simulink model "modelo2a"  (R2024b)
settings: Solver=ode4  StartTime=0.0  StopTime=t_final  FixedStep=t_step  RelTol=1e-3  EnableMultiTasking=on
InitFcn:
  | modelo2Initialization
undefined symbols (not defined in the file): Earth, IC, Quadrotor, sigbuilder_block, t_step, WGS84
libraries: simulink_extras x2, aerolibfltsims x2, aerolibobsolete x1, aerolibtransform2 x1, aerolibanimutils x1
settings Model: Creator=claus  LastModifiedBy=krish
settings SolverCC: ShapePreserveControl=EnableAll  AlgebraicLoopSolver=TrustRegion
settings DataIOCC: LimitDataPoints=on  SaveFormat=Array  ReturnWorkspaceOutputs=off
settings OptimizationCC: ExpressionDepthLimit=2147483647  EfficientMapNaN2IntZero=off  LifeSpan=inf  SimCompilerOptimization=on  AccelVerboseBuild=on
settings DebuggingCC: UnderspecifiedInitializationDetection=Classic  MergeDetectMultiDrivingBlocksExec=none  SolverPrmCheckMsg=warning  UnconnectedInputMsg=warning  UnconnectedOutputMsg=warning  UnconnectedLineMsg=warning  StateNameClashWarn=warning  SFUnexpectedBacktrackingDiag=warning  SFNoUnconditionalDefaultTransitionDiag=warning  SFExecutionAtInitializationDiag=none  ArithmeticOperatorsInVariantConditions=warning
settings HardwareCC: ProdBitPerPointer=32  ProdBitPerSizeT=32  ProdBitPerPtrDiffT=32  ProdLargestAtomicFloat=None  ProdIntDivRoundTo=Undefined  ProdEndianess=Unspecified  ProdWordSize=32  ProdHWDeviceType=32-bit Generic  TargetBitPerPointer=64  TargetBitPerSizeT=64  TargetBitPerPtrDiffT=64  TargetLongLongMode=on  TargetIntDivRoundTo=Zero  TargetEndianess=LittleEndian  TargetWordSize=64  TargetHWDeviceType=MATLAB Host  ProdEqTarget=off
settings ModelReferenceCC: EnableParallelModelReferenceBuilds=on  PropagateSignalLabelsOutOfModel=off
settings SFSimCC: SimUseLocalCustomCode=off  CustomCodeUndefinedFunction=UseInterfaceOnly
settings RTWCC: RTWUseLocalCustomCode=off  GPUComputeCapability=3.5
settings CodeAppCC: MaxIdLength=128  StateflowObjectComments=on
settings GRTTargetCC: TargetLangStandard=C89/C90 (ANSI)  CombineOutputUpdateFcns=off  GRTInterface=on
settings ConfigComp: CovMetricSettings=dw  CovSaveCumulativeToWorkspaceVar=on  CovSaveSingleToWorkspaceVar=on  CovExternalEMLEnable=off

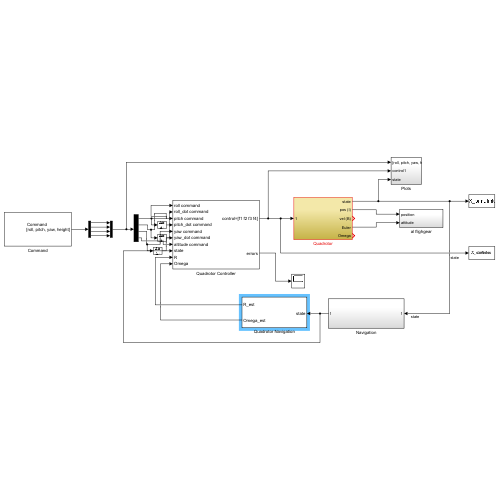
[thumbnail: Simulink's stored preview of the top-level diagram]
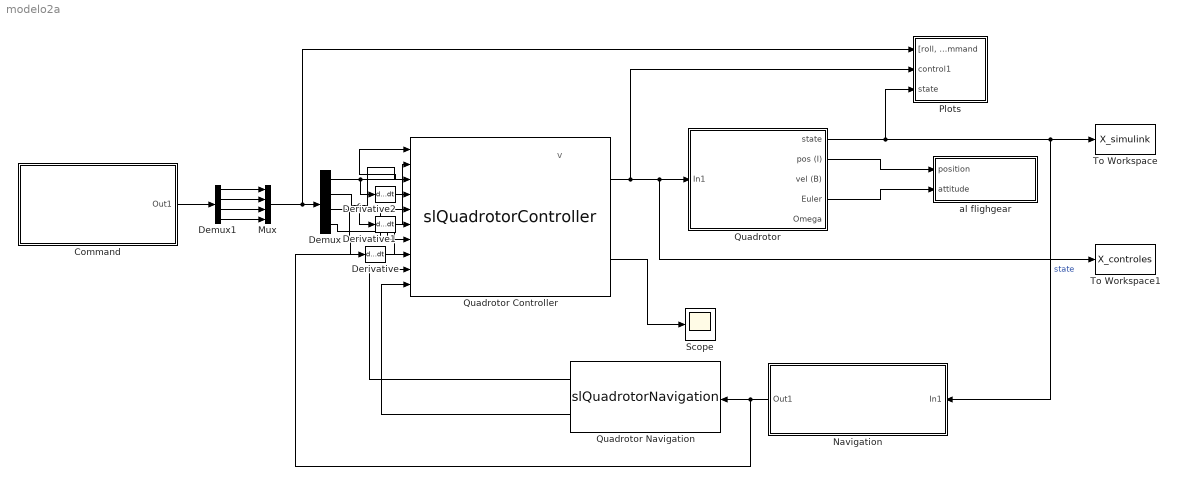
== system modelo2a ==
  note: v
  Command : Subsystem
      mask Display:
      | fprintf('Command \n \n')
      | port_label('output', 1, '[roll, pitch, yaw, height]')
  Demux : Demux
  Demux1 : Demux
  Derivative : Derivative
  Derivative1 : Derivative
  Derivative2 : Derivative
  Mux : Mux
  Navigation : Subsystem
  Plots : Subsystem
  Quadrotor : Subsystem
  Quadrotor Controller : M-S-Function  FunctionName=slQuadrotorController
      mask Display:
      | port_label('output', 1, 'control=[f1 f2 f3 f4]')
      | port_label('output', 2, 'errors')
      | port_label('input', 1, 'roll command')
      | port_label('input', 3, 'pitch command')
      | port_label('input', 5, 'yaw command')
      | port_label('input', 2, 'roll_dot command')
      | port_label('input', 4, 'pitch_dot command')
      | port_label('input', 6, 'yaw_dot command')
      | port_label('input', 7, 'altitude command')
      | port_label('input', 8, 'state')
      | port_label('input', 9, 'R')
      | port_label('input', 10, 'Omega')
  "Quadrotor Navigation " : M-S-Function  FunctionName=slQuadrotorNavigation
      mask Display:
      | port_label('output', 1, 'R_est')
      | port_label('output', 2, 'Omega_est')
      | port_label('input', 1, 'state')
  Scope : Scope
  To Workspace : ToWorkspace  VariableName=X_simulink  SaveFormat=Timeseries  SampleTime=-1
  To Workspace1 : ToWorkspace  VariableName=X_controles  SaveFormat=Timeseries  SampleTime=-1
  al flighgear : Subsystem
  wires:
  Quadrotor Controller/1 -> To Workspace1/1, Quadrotor/1(In1), Plots/2(control1)
  Quadrotor/1(state) -> Navigation/1(In1), To Workspace/1, Plots/3(state)  "state"
  Quadrotor/2(pos (I)) -> al flighgear/1(position)
  Quadrotor/4(Euler) -> al flighgear/2(attitude)
  Mux/1 -> Demux/1, Plots/1("[roll, pitch, yaw, height] command")
  Demux/1 -> Derivative2/1, Quadrotor Controller/1
  Demux/2 -> Derivative1/1, Quadrotor Controller/3
  Demux/3 -> Derivative/1, Quadrotor Controller/5
  Demux/4 -> Quadrotor Controller/7
  Derivative/1 -> Quadrotor Controller/6
  Derivative1/1 -> Quadrotor Controller/4
  Derivative2/1 -> Quadrotor Controller/2
  Command/1(Out1) -> Demux1/1
  Demux1/2 -> Mux/2
  "Quadrotor Navigation "/1 -> Quadrotor Controller/9
  "Quadrotor Navigation "/2 -> Quadrotor Controller/10
  Navigation/1(Out1) -> Quadrotor Controller/8, "Quadrotor Navigation "/1
  Quadrotor Controller/2 -> Scope/1
  Demux1/1 -> Mux/1
  Demux1/4 -> Mux/4
  Demux1/3 -> Mux/3

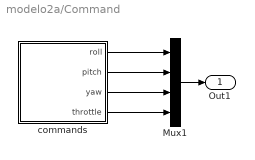
== system modelo2a/Command ==
  Mux1 : Mux
  commands : Subsystem  Tag=STV Subsys  LoadFcn=sigbuilder_block('load',[0 36 960 449.5 ]);  StartFcn=sigbuilder_block('start');  StopFcn=sigbuilder_block('stop');  ClipboardFcn=sigbuilder_block('clipboard');  mask(Sigbuilder block){tuvar=[0:10]}
      mask help: Simulink:masks:SigbuilderBlock_MD
      mask init:
      | if ~strcmp(get_param(bdroot(gcbh),'SimulationStatus'),'stopped') tuvar = sigbuilder_block('maskInit'); end
      settings: CopyFcn=sigbuilder_block('copy');  DeleteFcn=sigbuilder_block('delete');  ModelCloseFcn=sigbuilder_block('modelClose');  PreSaveFcn=sigbuilder_block('preSave');  PauseFcn=sigbuilder_block('pause');  ContinueFcn=sigbuilder_block('continue');  NameChangeFcn=sigbuilder_block('namechange');  OpenFcn=sigbuilder_block('open',[110.618 111.614 951.71 513.226 ]);  CloseFcn=sigbuilder_block('close');
      mask Display: plot(0, 0, 100, 100,[2, 2, 32, 32, 2], [68, 8, 8, 68, 68],[32, 2], [38, 38], [32, 19, 2],[53, 60, 44], [32, 17, 17, 2],[16, 16, 31, 31]);txt = getActiveGroup(gcbh);text(2, 100, txt,'verticalAlignment', 'top');
  Out1 : Outport
  wires:
  commands/1(roll) -> Mux1/1
  commands/2(pitch) -> Mux1/2
  commands/3(yaw) -> Mux1/3
  commands/4(throttle) -> Mux1/4
  Mux1/1 -> Out1/1

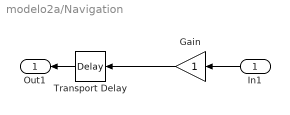
== system modelo2a/Navigation ==
  In1 : Inport
  Gain : Gain
  Transport Delay : TransportDelay  DelayTime=t_step*1
  Out1 : Outport
  wires:
  Gain/1 -> Transport Delay/1
  In1/1 -> Gain/1
  Transport Delay/1 -> Out1/1

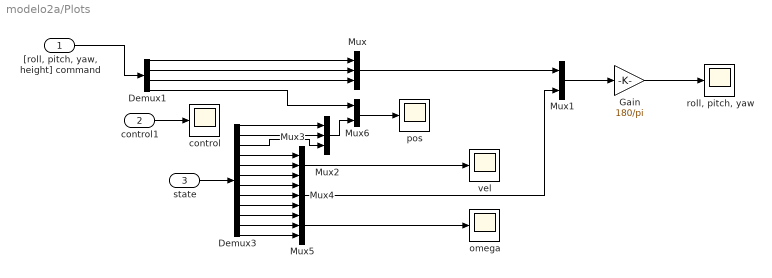
== system modelo2a/Plots ==
  "[roll, pitch, yaw, height] command" : Inport
  control1 : Inport  Port=2
  state : Inport  Port=3
  Demux1 : Demux
  Demux3 : Demux  Outputs=12
  Gain : Gain  Gain=180/pi
  Mux{,2..5} (5 alike) : Mux  Inputs=3
  Mux1 : Mux  Inputs=2
  Mux6 : Mux  Inputs=2
  control : Scope
  omega : Scope
  pos : Scope
  "roll, pitch, yaw" : Scope
  vel : Scope
  wires:
  Mux/1 -> Mux1/1
  Mux1/1 -> Gain/1
  Demux3/1 -> Mux2/1
  Demux3/2 -> Mux2/2
  Demux3/3 -> Mux2/3
  Demux3/4 -> Mux3/1
  Demux3/5 -> Mux3/2
  Demux3/6 -> Mux3/3
  Demux3/7 -> Mux4/1
  Demux3/8 -> Mux4/2
  Demux3/9 -> Mux4/3
  Demux3/10 -> Mux5/1
  Demux3/11 -> Mux5/2
  Demux3/12 -> Mux5/3
  Mux4/1 -> Mux1/2
  Mux6/1 -> pos/1
  Mux2/1 -> Mux6/2
  Mux5/1 -> omega/1
  Mux3/1 -> vel/1
  "[roll, pitch, yaw, height] command"/1 -> Demux1/1
  control1/1 -> control/1
  state/1 -> Demux3/1
  Demux1/4 -> Mux6/1
  Demux1/1 -> Mux/1
  Demux1/3 -> Mux/3
  Demux1/2 -> Mux/2
  Gain/1 -> "roll, pitch, yaw"/1

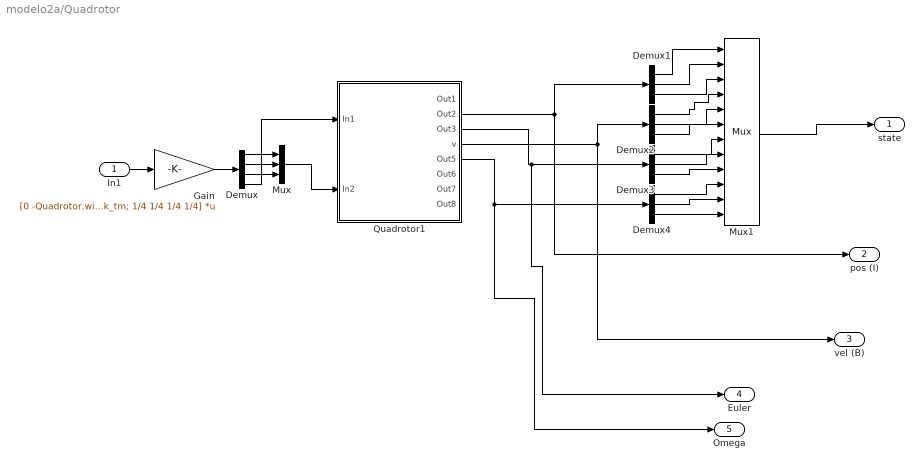
== system modelo2a/Quadrotor ==
  In1 : Inport
  Demux : Demux
  Demux{1..4} (4 alike) : Demux  Outputs=3
  Gain : Gain  Gain=[0 -Quadrotor.width/2 0 Quadrotor.width/2; -Quadrotor.width/2 0 Quadrotor.width/2 0; Quadrotor.k_tm -Quadrotor.k_tm Quadrotor.k_tm -Quadrotor.k_tm; 1/4 1/4 1/4 1/4]  Multiplication=Matrix(K*u)
  Mux : Mux  Inputs=3
  Mux1 : Mux  Inputs=12
  Quadrotor1 : Subsystem
      mask Display:
      | port_label('input', 1, 'Fz')
      | port_label('input', 2, 'Mxyz')
      | port_label('output', 2, 'r')
      | port_label('output', 3, 'Euler')
      | port_label('output', 4, 'v')
      | port_label('output', 5, 'Omega')
      | port_label('output', 8, 'R')
  state : Outport
  pos (I) : Outport  Port=2
  vel (B) : Outport  Port=3
  Euler : Outport  Port=4
  Omega : Outport  Port=5
  wires:
  Gain/1 -> Demux/1
  Mux/1 -> Quadrotor1/2(In2)
  Quadrotor1/4(v) -> vel (B)/1, Demux2/1
  Quadrotor1/3(Out3) -> Euler/1, Demux3/1
  Quadrotor1/5(Out5) -> Omega/1, Demux4/1
  Demux1/3 -> Mux1/3
  Demux1/2 -> Mux1/2
  Demux1/1 -> Mux1/1
  Demux2/1 -> Mux1/4
  Demux2/2 -> Mux1/5
  Demux2/3 -> Mux1/6
  Demux3/1 -> Mux1/7
  Demux3/2 -> Mux1/8
  Demux3/3 -> Mux1/9
  Demux4/1 -> Mux1/10
  Demux4/2 -> Mux1/11
  Demux4/3 -> Mux1/12
  Mux1/1 -> state/1
  Quadrotor1/2(Out2) -> pos (I)/1, Demux1/1
  In1/1 -> Gain/1
  Demux/2 -> Mux/2
  Demux/3 -> Mux/3
  Demux/1 -> Mux/1
  Demux/4 -> Quadrotor1/1(In1)

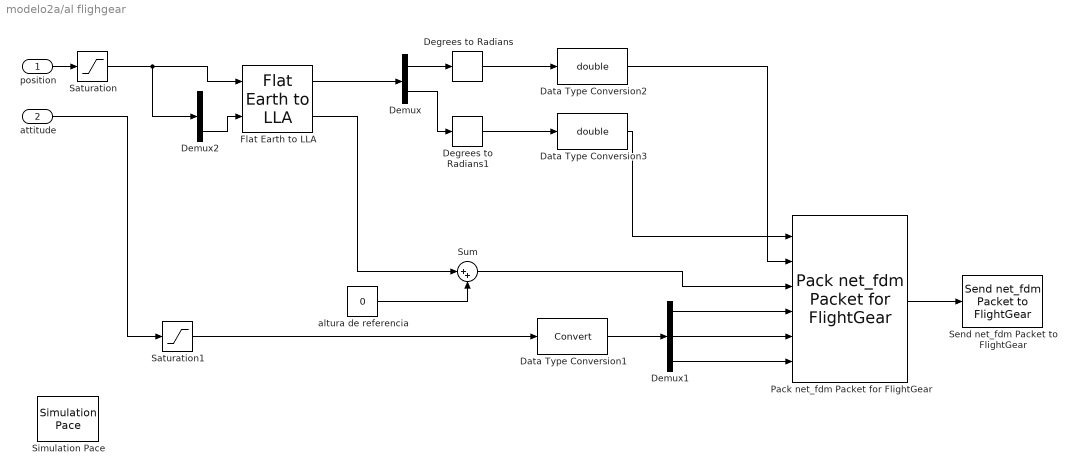
== system modelo2a/al flighgear ==
  position : Inport
  attitude : Inport  Port=2
  Data Type Conversion1 : DataTypeConversion  SaturateOnIntegerOverflow=off  RndMeth=Floor
  Data Type Conversion2 : DataTypeConversion  OutDataTypeStr=double  SaturateOnIntegerOverflow=off  RndMeth=Floor
  Data Type Conversion3 : DataTypeConversion  OutDataTypeStr=double  SaturateOnIntegerOverflow=off  RndMeth=Floor
  Degrees to Radians : simulink_extras/Transformations/Degrees to Radians
  Degrees to Radians1 : simulink_extras/Transformations/Degrees to Radians
  Demux : Demux  Outputs=2
  Demux1 : Demux  Outputs=3
  Demux2 : Demux  Outputs=3
  Flat Earth to LLA : aerolibtransform2/Flat Earth to LLA  units=Metric (MKS)  ptype=Earth (WGS84)  F=1/298.257223563  R=6378137  refPosPort=off  LL0=IC.LatLonAltOnEarth(1:2)  psi=0
  Pack net_fdm Packet for FlightGear : aerolibfltsims/Pack net_fdm Packet for FlightGear  FlightGearVersion=v2.8  ShowPositionAttitudeInputs=on  ShowVelocityAccelerationInputs=off  ShowControlSurfacePositionInputs=off  ShowEngineFuelInputs=off  ShowLandingGearInputs=off  ShowEnvironmentInputs=off  SampleTime=-1  packetVersion=24
  Saturation : Saturate  UpperLimit=100  LowerLimit=-100
  Saturation1 : Saturate  UpperLimit=100  LowerLimit=-100
  Send net_fdm Packet to FlightGear : aerolibfltsims/Send net_fdm Packet to FlightGear  DestinationIpAddress=127.0.0.1  DestinationPort=5502  LocalIpPort=-1  varLen=off  SampleTime=-1
  Simulation Pace : aerolibanimutils/Simulation Pace  SimulationPace=1  SleepMode=MATLAB Thread  OutputPaceError=off  SampleTime=-1
      settings: AttributesFormatString=%<SimulationPace> sec/sec
  Sum : Sum  Inputs=|++
  altura de referencia : Constant  Value=0
  wires:
  position/1 -> Saturation/1
  attitude/1 -> Saturation1/1
  Pack net_fdm Packet for FlightGear/1 -> Send net_fdm Packet to FlightGear/1
  Demux1/1 -> Pack net_fdm Packet for FlightGear/4
  Demux1/2 -> Pack net_fdm Packet for FlightGear/5
  Demux1/3 -> Pack net_fdm Packet for FlightGear/6
  Data Type Conversion1/1 -> Demux1/1
  Flat Earth to LLA/1 -> Demux/1
  Demux2/3 -> Flat Earth to LLA/2
  Degrees to Radians/1 -> Data Type Conversion2/1
  Degrees to Radians1/1 -> Data Type Conversion3/1
  Demux/1 -> Degrees to Radians/1
  Demux/2 -> Degrees to Radians1/1
  Data Type Conversion3/1 -> Pack net_fdm Packet for FlightGear/1
  Data Type Conversion2/1 -> Pack net_fdm Packet for FlightGear/2
  Flat Earth to LLA/2 -> Sum/1
  altura de referencia/1 -> Sum/2
  Sum/1 -> Pack net_fdm Packet for FlightGear/3
  Saturation/1 -> Demux2/1, Flat Earth to LLA/1
  Saturation1/1 -> Data Type Conversion1/1

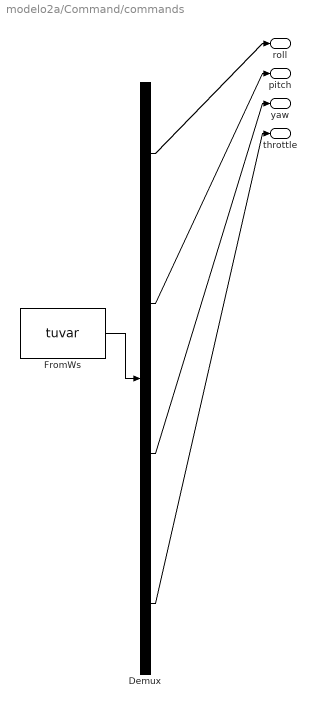
== system modelo2a/Command/commands ==
  Demux : Demux  Tag=STV Demux
      settings: DisplayOption=none
  FromWs : FromWorkspace  Tag=STV FromWs  VariableName=tuvar
      SigBuilderData=|
      | common.afterFinalStr = 'Extrapolate'
      | common.sampleTime = 0
      | dataSet.timeRange = [0 15]
      | dataSet.name = 'Group 1'
      | sbobj.Groups.Name = 'Group 1'
      | sbobj.Groups.Signals(1).Name = 'roll'
      | sbobj.Groups.Signals(1).XData = [0 1 2 2 6 6 7 11 12 15]
      | sbobj.Groups.Signals(1).YData = [0 0 6.28 6.3 6.3 6.28 -0.3 -0.3 0 0]
      | sbobj.Groups.Signals(2).Name = 'pitch'
      | sbobj.Groups.Signals(2).XData = [0 1 5 11.4 15]
      | sbobj.Groups.Signals(2).YData = [0 0 0 0 0]
      | sbobj.Groups.Signals(3).Name = 'yaw'
      | sbobj.Groups.Signals(3).XData = [0 0.6 3.45 5 6.5 8.5 15]
      | sbobj.Groups.Signals(3).YData = [0 0 0 0 0 0 0]
      | sbobj.Groups.Signals(4).Name = 'throttle'
      | sbobj.Groups.Signals(4).XData = [0 0.94 1 2.94 2.94 5.8 5.8 11.1 11.1 15]
      | sbobj.Groups.Signals(4).YData = [7.4 22 0 0 8.5 19 1.4 1.4 5 5]
      | sbobj.Groups.TimeRange = [0 15]
  roll : Outport  Tag=STV Outport
  pitch : Outport  Tag=STV Outport  Port=2
  yaw : Outport  Tag=STV Outport  Port=3
  throttle : Outport  Tag=STV Outport  Port=4
  wires:
  FromWs/1 -> Demux/1
  Demux/1 -> roll/1
  Demux/2 -> pitch/1
  Demux/3 -> yaw/1
  Demux/4 -> throttle/1

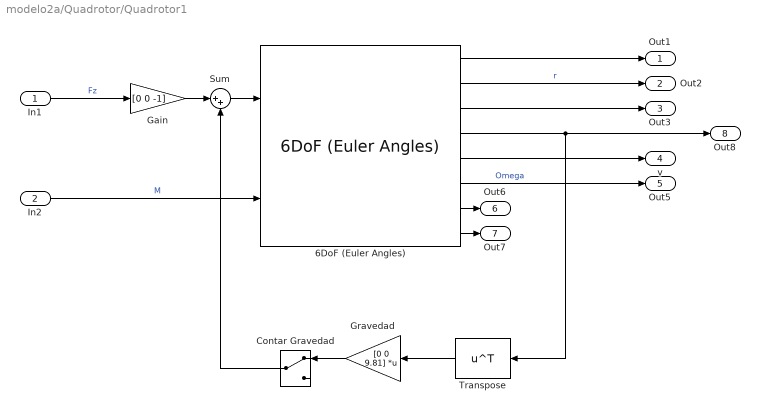
== system modelo2a/Quadrotor/Quadrotor1 ==
  In1 : Inport
  In2 : Inport  Port=2
  6DoF (Euler Angles) : aerolibobsolete/6DoF (Euler Angles)  units=Metric (MKS)  mtype=Fixed  rep=Euler Angles  xme_0=IC.position  Vm_0=[0 0 0]  eul_0=[0 0 0]  pm_0=[0 0 0]  mass_0=Quadrotor.Mass_prop.Mass  mass_e=0.5  mass_f=2.0  inertia=Quadrotor.Mass_prop.I  inertia_e=eye(3)  inertia_f=2*eye(3)  k_quat=1.0
  Contar Gravedad : ManualSwitch
  Gain : Gain  Gain=[0 0 -1]
  Gravedad : Gain  Gain=[0 0 9.81]  Multiplication=Matrix(K*u)
  Sum : Sum  Inputs=|++
  Transpose : Math  Operator=transpose
  Out1 : Outport
  Out2 : Outport  Port=2
  Out3 : Outport  Port=3
  v : Outport  Port=4
  Out5 : Outport  Port=5
  Out6 : Outport  Port=6
  Out7 : Outport  Port=7
  Out8 : Outport  Port=8
  wires:
  6DoF (Euler Angles)/5 -> v/1
  6DoF (Euler Angles)/3 -> Out3/1
  6DoF (Euler Angles)/8 -> Out7/1
  6DoF (Euler Angles)/7 -> Out6/1
  6DoF (Euler Angles)/1 -> Out1/1
  In1/1 -> Gain/1  "Fz"
  In2/1 -> 6DoF (Euler Angles)/2  "M"
  6DoF (Euler Angles)/2 -> Out2/1  "r"
  6DoF (Euler Angles)/6 -> Out5/1  "Omega"
  6DoF (Euler Angles)/4 -> Transpose/1, Out8/1
  Gain/1 -> Sum/1
  Sum/1 -> 6DoF (Euler Angles)/1
  Contar Gravedad/1 -> Sum/2
  Transpose/1 -> Gravedad/1
  Gravedad/1 -> Contar Gravedad/1
